simulink model "ADC_reader_simulink (1)"  (R2025a)
settings: Solver=FixedStepAuto  StartTime=0.0  StopTime=10  FixedStep=0.01  RelTol=1e-3  EnableMultiTasking=on
libraries: stm32f4xxblockslib x8
settings Model: STM32="{\"AnalogInput\":[{\"ID\":\"test_poten:20\"},{\"ID\":\"test_poten:28\"},{\"ID\":\"ADC_reader:28\"},{\"ID\":\"ADC_reader:20\"},{\"ID\":\"ADC_reader:14\"},{\"ID\":\"ADC_reader:11\"},{\"ID\":\"ADC_reader:8\"},{\"ID\":\"ADC_reader:5\"},{\"ID\":\"ADC_reader:1\"},{\"ID\":\"ADC_reader_simulink:5\"},{\"ID\":\"ADC_reader_simulink:8\"},{\"ID\":\"ADC_reader_simulink:11\"},{\"ID\":\"ADC_reader_simulink:14\"},{\"ID\":\"ADC_reader_simulink:28\"},{\"ID\":\"ADC_reader_simulink:37\"},{\"ID\":\"ADC_reader_simulink:20\"}]}"  Creator=ioonz  LastModifiedBy=User
settings OptimizationCC: DefaultParameterBehavior=Inlined  EnhancedBackFolding=on  PassReuseOutputArgsAs=Individual arguments  ZeroExternalMemoryAtStartup=off  ZeroInternalMemoryAtStartup=off  MaxStackSize=512  OptimizeBlockOrder=speed  DifferentSizesBufferReuse=on  OptimizationCustomize=off  EfficientTunableParamExpr=on
settings DebuggingCC: ParameterTunabilityLossMsg=error
settings HardwareCC: ProdBitPerPointer=32.0  ProdBitPerSizeT=32.0  ProdBitPerPtrDiffT=32.0  ProdLargestAtomicInteger=Long  ProdLargestAtomicFloat=Double  ProdWordSize=32.0  ProdLongLongMode=on  ProdHWDeviceType=ARM Compatible->ARM Cortex-M
settings SFSimCC: MATLABDynamicMemAlloc=off
settings RTWCC: SystemTargetFile=ert.tlc  HardwareBoard=STM32G4xx Based  TemplateMakefile=ert_default_tmf  Toolchain=GNU Tools for ARM Embedded Processors  Description=Embedded Coder
settings CodeAppCC: ForceParamTrailComments=on  IgnoreCustomStorageClasses=off  OperatorAnnotations=on  SimulinkDataObjDesc=on  SFDataObjDesc=on  InsertBlockDesc=on
settings ERTTargetCC: ExtModeTransport=3.0  ExtModeStaticAllocSize=2048.0  TargetLangStandard=C99 (ISO)  CodeReplacementLibrary=ARM Cortex-M

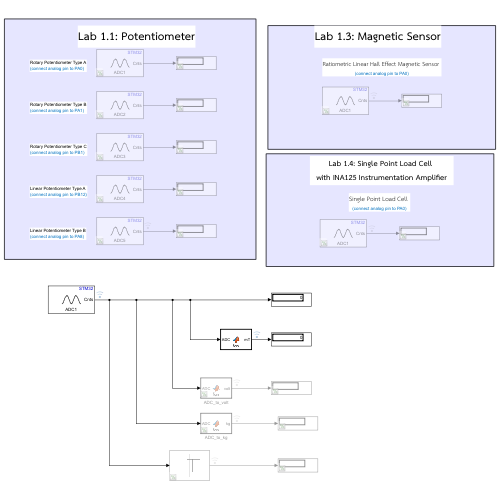
[thumbnail: Simulink's stored preview of the top-level diagram]
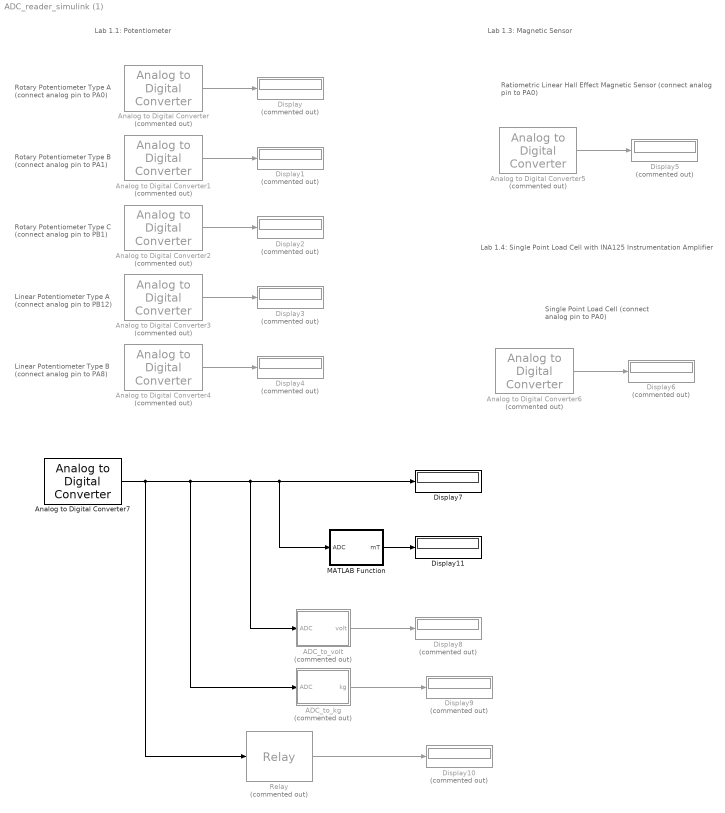
== system ADC_reader_simulink (1) ==
  note: Lab 1.1: Potentiometer
  note: Rotary Potentiometer Type A
      | (connect analog pin to PA0)
  note: Rotary Potentiometer Type B
      | (connect analog pin to PA1)
  note: Rotary Potentiometer Type C
      | (connect analog pin to PB1)
  note: Linear Potentiometer Type A
      | (connect analog pin to PB12)
  note: Linear Potentiometer Type B
      | (connect analog pin to PA8)
  note: Ratiometric Linear Hall Effect Magnetic Sensor
      | (connect analog pin to PA0)
  note: Single Point Load Cell
      | (connect analog pin to PA0)
  note: Lab 1.3: Magnetic Sensor
  note: Lab 1.4: Single Point Load Cell
      | with INA125 Instrumentation Amplifier
  ADC_to_kg : MATLAB Function  Commented=on  TreatAsAtomicUnit=on
  ADC_to_volt : MATLAB Function  Commented=on  TreatAsAtomicUnit=on
  Analog to Digital Converter : stm32f4xxblockslib/Analog to Digital Converter  Commented=on  ADCModule=ADC1  ConversionGroup=Regular  TriggerMode=Trigger and read  NumberOfConversions=1  EnableBufferConv=off  BufferLength=1  OutputStatus=off  SampleTime=-1  EnableSimPort=off  hoistedMaskSrc=ECSoC/ECSimCodegen/Analog to Digital Converter
  Analog to Digital Converter1 : stm32f4xxblockslib/Analog to Digital Converter  Commented=on  ADCModule=ADC2  ConversionGroup=Regular  TriggerMode=Trigger and read  NumberOfConversions=1  EnableBufferConv=off  BufferLength=1  OutputStatus=off  SampleTime=-1  EnableSimPort=off  hoistedMaskSrc=ECSoC/ECSimCodegen/Analog to Digital Converter
  Analog to Digital Converter2 : stm32f4xxblockslib/Analog to Digital Converter  Commented=on  ADCModule=ADC3  ConversionGroup=Regular  TriggerMode=Trigger and read  NumberOfConversions=1  EnableBufferConv=off  BufferLength=1  OutputStatus=off  SampleTime=-1  EnableSimPort=off  hoistedMaskSrc=ECSoC/ECSimCodegen/Analog to Digital Converter
  Analog to Digital Converter3 : stm32f4xxblockslib/Analog to Digital Converter  Commented=on  ADCModule=ADC4  ConversionGroup=Regular  TriggerMode=Trigger and read  NumberOfConversions=1  EnableBufferConv=off  BufferLength=1  OutputStatus=off  SampleTime=-1  EnableSimPort=off  hoistedMaskSrc=ECSoC/ECSimCodegen/Analog to Digital Converter
  Analog to Digital Converter4 : stm32f4xxblockslib/Analog to Digital Converter  Commented=on  ADCModule=ADC5  ConversionGroup=Regular  TriggerMode=Trigger and read  NumberOfConversions=1  EnableBufferConv=off  BufferLength=1  OutputStatus=off  SampleTime=-1  EnableSimPort=off  hoistedMaskSrc=ECSoC/ECSimCodegen/Analog to Digital Converter
  Analog to Digital Converter5 : stm32f4xxblockslib/Analog to Digital Converter  Commented=on  ADCModule=ADC1  ConversionGroup=Regular  TriggerMode=Trigger and read  NumberOfConversions=1  EnableBufferConv=off  BufferLength=1  OutputStatus=off  SampleTime=-1  EnableSimPort=off  hoistedMaskSrc=ECSoC/ECSimCodegen/Analog to Digital Converter
  Analog to Digital Converter6 : stm32f4xxblockslib/Analog to Digital Converter  Commented=on  ADCModule=ADC1  ConversionGroup=Regular  TriggerMode=Trigger and read  NumberOfConversions=1  EnableBufferConv=off  BufferLength=1  OutputStatus=off  SampleTime=-1  EnableSimPort=off  hoistedMaskSrc=ECSoC/ECSimCodegen/Analog to Digital Converter
  Analog to Digital Converter7 : stm32f4xxblockslib/Analog to Digital Converter  ADCModule=ADC1  ConversionGroup=Regular  TriggerMode=Trigger and read  NumberOfConversions=1  EnableBufferConv=off  BufferLength=1  OutputStatus=off  SampleTime=-1  EnableSimPort=off  hoistedMaskSrc=ECSoC/ECSimCodegen/Analog to Digital Converter
  Display{,1..6,8..10} (10 alike) : Display  Commented=on
  Display11 : Display
  Display7 : Display
  MATLAB Function : MATLAB Function  TreatAsAtomicUnit=on
  Relay : Relay  Commented=on  OnSwitchValue=3071.25  OffSwitchValue=1023.75
  wires:
  Analog to Digital Converter/1 -> Display/1
  Analog to Digital Converter1/1 -> Display1/1
  Analog to Digital Converter2/1 -> Display2/1
  Analog to Digital Converter3/1 -> Display3/1
  Analog to Digital Converter4/1 -> Display4/1
  Analog to Digital Converter5/1 -> Display5/1
  Analog to Digital Converter6/1 -> Display6/1
  ADC_to_volt/1(volt) -> Display8/1
  ADC_to_kg/1(kg) -> Display9/1
  Analog to Digital Converter7/1 -> Relay/1, ADC_to_kg/1(ADC), ADC_to_volt/1(ADC), MATLAB Function/1(ADC), Display7/1
  Relay/1 -> Display10/1
  MATLAB Function/1(mT) -> Display11/1

== matlab function ADC_reader_simulink (1)/ADC_to_volt ==
  data: ADC input; volt output
function volt = fcn(ADC)
ADC_double=double(ADC);
volt = (ADC_double/4045.00)*3.3;

== matlab function ADC_reader_simulink (1)/MATLAB Function ==
  data: ADC input; mT output
function mT = fcn(ADC)

Vq=((4095/2)/4095)*3.3*1000;
Sensitivity=60;
 mT=(((ADC/4095)*3.3*1000)-Vq)/Sensitivity;

== matlab function ADC_reader_simulink (1)/ADC_to_kg ==
  data: ADC input; kg output
function kg = fcn(ADC)

ADC_input_double=double(ADC);
max_kg=10.008;
min_kg=0;
max_measure_volt=2.44;
min_measure_volt=0.1;
max_measure_ADC=(max_measure_volt*4095)/3.3;
min_measure_ADC=(min_measure_volt*4095)/3.3;
ADC_offset=125;
% convert ADC to kg
map_scale=(max_kg-min_kg)/(max_measure_ADC-min_measure_ADC);

kg=(ADC_input_double-ADC_offset)*map_scale;
